simulink model "stanleyController"  (R2022b)
settings: Solver=VariableStepAuto  StartTime=0.0  StopTime=inf  FixedStep=0.001  RelTol=1e-3
PreLoadFcn:
  | setUpModel
  | close
model workspace (MAT data in the model file):
  firstWarning = 0
  originalScenarioChecksum = 'F73A6DA3C723D3CA73A6F931B7A52A9C'
undefined symbols (not defined in the file or in its folder): Angular, direction, esc, hz, Linear, path
libraries: robotlib x4, drivingvehiclecontroller x1, dspstat3 x1
settings Model: PacingRate=0.500000  Creator=valakshe  LastModifiedBy=kishor
settings SolverCC: AlgebraicLoopSolver=TrustRegion
settings DebuggingCC: UnconnectedInputMsg=warning  UnconnectedOutputMsg=warning  UnconnectedLineMsg=warning  SFMachineParentedDataDiag=warning
settings ModelReferenceCC: EnableRefExpFcnMdlSchedulingChecks=on
settings RTWCC: DLArmComputeVersion=19.05

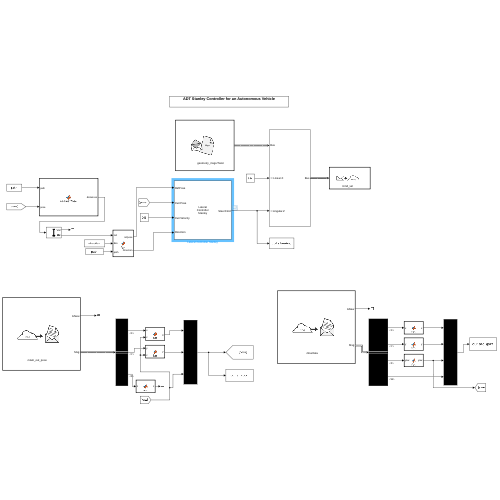
[thumbnail: Simulink's stored preview of the top-level diagram]
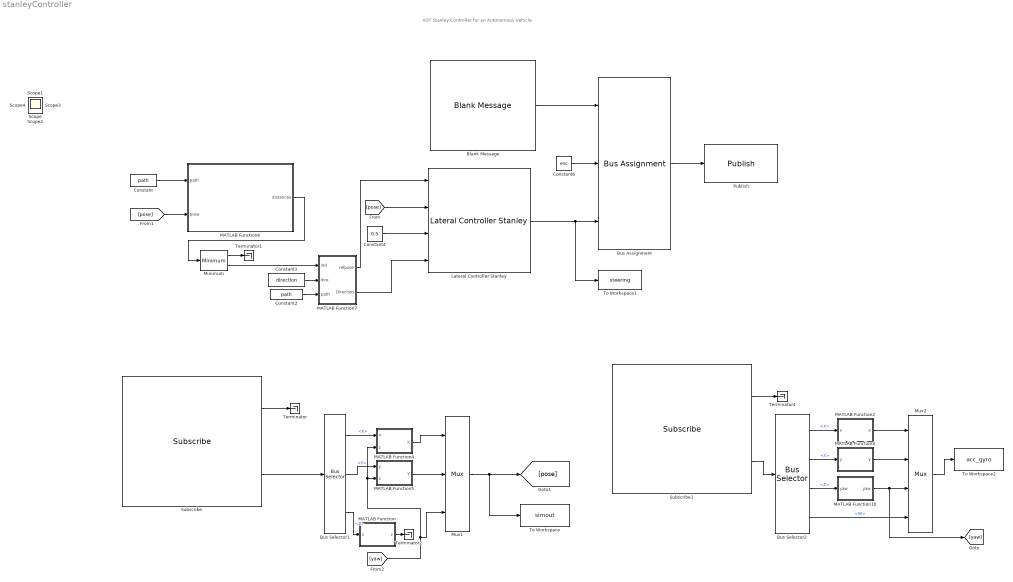
== system stanleyController ==
  note: ADT Stanley Controller for an Autonomous Vehicle
  Blank Message : robotlib/Blank Message  messageClass=Message  entityType=geometry_msgs/Twist  messageType=geometry_msgs/Twist  SampleTime=1/hz  legacyBusStruct=off
      settings: LibrarySourceBlock=roslib/ROS/Blank Message
  Bus Assignment : BusAssignment  AssignedSignals=Linear.X,Angular.Z
  Bus Selector1 : BusSelector  OutputSignals=Pose.Position.X,Pose.Position.Y,Pose.Orientation.Z
  Bus Selector2 : BusSelector  OutputSignals=LinearAcceleration.X,LinearAcceleration.Y,Orientation.Z,Orientation.W
  Constant : Constant  Value=path  SampleTime=1/hz
  Constant1 : Constant  Value=direction  SampleTime=1/hz
  Constant2 : Constant  Value=path  SampleTime=1/hz
  Constant4 : Constant  Value=0.5
  Constant6 : Constant  Value=esc  SampleTime=1/hz
  Lateral Controller Stanley : drivingvehiclecontroller/Lateral Controller Stanley  ModelType=Kinematic bicycle model  PositionGainF=K  PositionGainR=K  YawRateGain=0.2  DelayGain=0.2  VehicleMass=1970  Lf=1.11  Lr=1.67  TireStiffness=83540  Wheelbase=0.330  MaxSteeringAngle=30
  MATLAB Function : MATLAB Function  TreatAsAtomicUnit=on
  MATLAB Function10 : MATLAB Function  TreatAsAtomicUnit=on
  MATLAB Function2 : MATLAB Function  TreatAsAtomicUnit=on
  MATLAB Function3 : MATLAB Function  TreatAsAtomicUnit=on
  MATLAB Function4 : MATLAB Function  TreatAsAtomicUnit=on
  MATLAB Function5 : MATLAB Function  TreatAsAtomicUnit=on
  MATLAB Function6 : MATLAB Function  TreatAsAtomicUnit=on
  MATLAB Function7 : MATLAB Function  TreatAsAtomicUnit=on
  Minimum : dspstat3/Minimum  operation=minimum  fcn=Value and Index  indexBase=One  operateOver=Each row  Dimension=1  InputProcessing=Columns as channels (frame based)  reset=None  roiEnable=off  roiType=Rectangles  roiPortion=Entire ROI  roiOutput=Individual statistics for each ROI  roiFlag=off  roundingMode=Floor  overflowMode=off
  Mux1 : Mux  Inputs=3
  Mux2 : Mux
  Publish : robotlib/Publish  topicSource=Specify your own  topic=/cmd_vel  messageType=geometry_msgs/Twist  legacyBusStruct=off  messageQueueLength=1
      settings: LibrarySourceBlock=roslib/ROS/Publish
  Subscribe : robotlib/Subscribe  topicSource=Specify your own  topic=/slam_out_pose  messageType=geometry_msgs/PoseStamped  SampleTime=1/hz  legacyBusStruct=off  messageQueueLength=1
      settings: LibrarySourceBlock=roslib/ROS/Subscribe
  Subscribe1 : robotlib/Subscribe  topicSource=Specify your own  topic=/imu/data  messageType=sensor_msgs/Imu  SampleTime=1/hz  legacyBusStruct=off  messageQueueLength=1
      settings: LibrarySourceBlock=roslib/ROS/Subscribe
  Terminator{,1..2,4} (4 alike) : Terminator
  To Workspace : ToWorkspace  VariableName=simout  SaveFormat=Timeseries  SampleTime=-1
  To Workspace1 : ToWorkspace  VariableName=steering  SaveFormat=Structure With Time  SampleTime=-1
  To Workspace2 : ToWorkspace  VariableName=acc_gyro  SaveFormat=Structure With Time  SampleTime=-1
  Scope{,1..4} (5 alike) : Scope
  wires:
  [pose] -> Lateral Controller Stanley/2
  Constant6/1 -> Bus Assignment/2
  Bus Assignment/1 -> Publish/1
  Blank Message/1 -> Bus Assignment/1
  Constant4/1 -> Lateral Controller Stanley/3
  [pose] -> MATLAB Function6/2(pose)
  Constant/1 -> MATLAB Function6/1(path)
  MATLAB Function6/1(distances) -> Minimum/1
  Constant1/1 -> MATLAB Function7/2(dire)
  MATLAB Function7/2(Direction) -> Lateral Controller Stanley/4
  Minimum/2 -> MATLAB Function7/1(ind)
  Constant2/1 -> MATLAB Function7/3(path)
  MATLAB Function7/1(refpose) -> Lateral Controller Stanley/1
  Minimum/1 -> Terminator1/1
  [yaw] -> MATLAB Function5/2(z), MATLAB Function4/2(z), Mux1/3
  Mux2/1 -> To Workspace2/1
  Bus Selector1/1 -> MATLAB Function4/1(x)  "<X>"
  Subscribe1/1 -> Terminator4/1
  Bus Selector1/3 -> MATLAB Function/1("z ")  "<Z>"
  Mux1/1 -> [pose], To Workspace/1
  Bus Selector2/1 -> MATLAB Function2/1("x ")  "<X>"
  MATLAB Function/1(z) -> Terminator2/1
  Subscribe/2 -> Bus Selector1/1
  MATLAB Function5/1(Y) -> Mux1/2
  Bus Selector2/2 -> MATLAB Function3/1("y ")  "<Y>"
  MATLAB Function10/1(yaw) -> [yaw], Mux2/3
  MATLAB Function3/1(y) -> Mux2/2
  Subscribe/1 -> Terminator/1
  MATLAB Function4/1(X) -> Mux1/1
  Bus Selector1/2 -> MATLAB Function5/1(y)  "<Y>"
  Bus Selector2/3 -> MATLAB Function10/1("yaw ")  "<Z>"
  Subscribe1/2 -> Bus Selector2/1
  Bus Selector2/4 -> Mux2/4  "<W>"
  MATLAB Function2/1(x) -> Mux2/1
  Lateral Controller Stanley/1 -> To Workspace1/1, Bus Assignment/3

== matlab function stanleyController/MATLAB Function ==
  data: z input; z output
function z = fcn(z)
z = z*180;
if (z < 0)
    z = 180 + (180 +z);
else
end
end

== matlab function stanleyController/MATLAB Function10 ==
  data: yaw input; yaw output
function yaw = fcn(yaw)
yaw = 360-yaw;
yaw = yaw*pi/180;
end

== matlab function stanleyController/MATLAB Function2 ==
  data: x input; x output
function x = fcn(x)
x = x - (0);
end

== matlab function stanleyController/MATLAB Function4 ==
  data: x input; X output; z input
function X = fcn(x,z)

X = x + 0.330*cos(z);

end

== matlab function stanleyController/MATLAB Function5 ==
  data: y input; Y output; z input
function Y = fcn(y,z)
Y = y + 0.330*sin(z);
end

== matlab function stanleyController/MATLAB Function6 ==
  data: path input; distances output; pose input
function distances  = nearestPose(path, pose)
    % path: Nx3 matrix containing the x, y, and heading of the waypoints in the path
    % current_pose: 1x3 vector containing the x, y, and heading of the current pose of the vehicle
    % nearest_pose: 1x3 vector containing the x, y, and heading of the nearest pose on the path
    % nearest_index: index of the nearest pose on the path
    
    % Find the distance from the current pose to each waypoint on the path
    
    l = length(path(:,1));
    cx = path(:,1);
    cy = path(:,2);
    cy = path(:,3);
    dx = zeros(1,l);
    dy = zeros(1,l);
    distances =  zeros(1,l);


    for i = 1:l
        dx(i) = pose(1) - cx(i);
        dy(i) = pose(2) - cy(i);
        distances(i) = sqrt((dx(i)^2+dy(i)^2));
    end
end

== matlab function stanleyController/MATLAB Function7 ==
  data: refpose output; ind input; dire input; Direction output; path input
function [refpose,Direction]= fcn(ind,dire,path)

Direction = dire(ind);
refpose = path(ind,:);
end

== matlab function stanleyController/MATLAB Function3 ==
  data: y input; y output
function y = fcn(y)
y = y - (0);
end
